simulink model "model_smpl"  (R2015a)
settings: Solver=ode45  StartTime=0.0  StopTime=Tfin  RelTol=1e-3
model workspace (MAT data in the model file):
  Sig = Simulink.Signal
  Sig.DataType = 'double'
  Sig.Dimensions = -1
  Sig.DimensionsMode = 'auto'
  Sig.Complexity = 'real'
  Sig.SampleTime = -1
  Sig.SamplingMode = 'auto'
  Sig.InitialValue = '[ ]'
values from neighbouring files (symbols this model uses):
  init_state = [ p_ini ]'    [main_parts.m]
  init_state_dot = [ 0 0 0 0 ]'    [main_parts.m]
undefined symbols (not defined in the file or in its folder): K, param, x, x_dot, x_r, y, y_dot, y_r
settings Model: Creator=jesus  LastModifiedBy=jesus

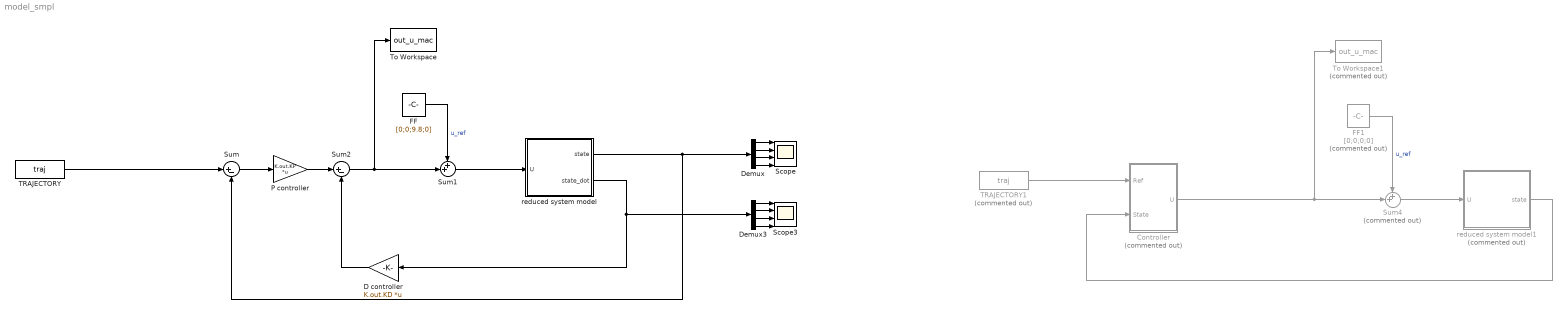
== system model_smpl ==
  Controller : Subsystem  Commented=on
  D controller : Gain  Gain=K.out.KD  Multiplication=Matrix(K*u)
  Demux : Demux
  Demux3 : Demux
  FF : Constant  Value=[0;0;9.8;0]
  FF1 : Constant  Commented=on  Value=[0;0;0;0]
  P controller : Gain  Gain=K.out.KP  Multiplication=Matrix(K*u)
  Scope : Scope  NumInputPorts=4
      settings: YMin=-5~-5~-5~-5  YMax=5~5~5~5
  Scope3 : Scope  NumInputPorts=4
      settings: YMin=-5~-5~-5~-5  YMax=5~5~5~5  SaveName=ScopeData3
  Sum : Sum  Inputs=|+-
  Sum1 : Sum  Inputs=++|
  Sum2 : Sum  Inputs=|+-
  Sum4 : Sum  Commented=on  Inputs=++|
  TRAJECTORY : FromWorkspace  VariableName=traj  SampleTime=param.hs  Interpolate=off  OutputAfterFinalValue=Setting to zero
  TRAJECTORY1 : FromWorkspace  Commented=on  VariableName=traj  SampleTime=param.hs  Interpolate=off  OutputAfterFinalValue=Setting to zero
  To Workspace : ToWorkspace  VariableName=out_u_mac  SaveFormat=Structure With Time  SampleTime=-1
  To Workspace1 : ToWorkspace  Commented=on  VariableName=out_u_mac  SaveFormat=Structure With Time  SampleTime=-1
  reduced system model : Subsystem
  reduced system model1 : Subsystem  Commented=on
  wires:
  Demux/1 -> Scope/1
  Demux/2 -> Scope/2
  Demux/3 -> Scope/3
  Demux/4 -> Scope/4
  Sum1/1 -> reduced system model/1(U)
  reduced system model/1(state) -> Sum/2, Demux/1
  FF/1 -> Sum1/1  "u_ref"
  Sum2/1 -> To Workspace/1, Sum1/2
  D controller/1 -> Sum2/2
  P controller/1 -> Sum2/1
  Sum/1 -> P controller/1
  TRAJECTORY/1 -> Sum/1
  Demux3/1 -> Scope3/1
  Demux3/2 -> Scope3/2
  Demux3/3 -> Scope3/3
  Demux3/4 -> Scope3/4
  reduced system model/2(state_dot) -> D controller/1, Demux3/1
  Sum4/1 -> reduced system model1/1(U)
  FF1/1 -> Sum4/1  "u_ref"
  TRAJECTORY1/1 -> Controller/1(Ref)
  reduced system model1/1(state) -> Controller/2(State)
  Controller/1(U) -> To Workspace1/1, Sum4/2

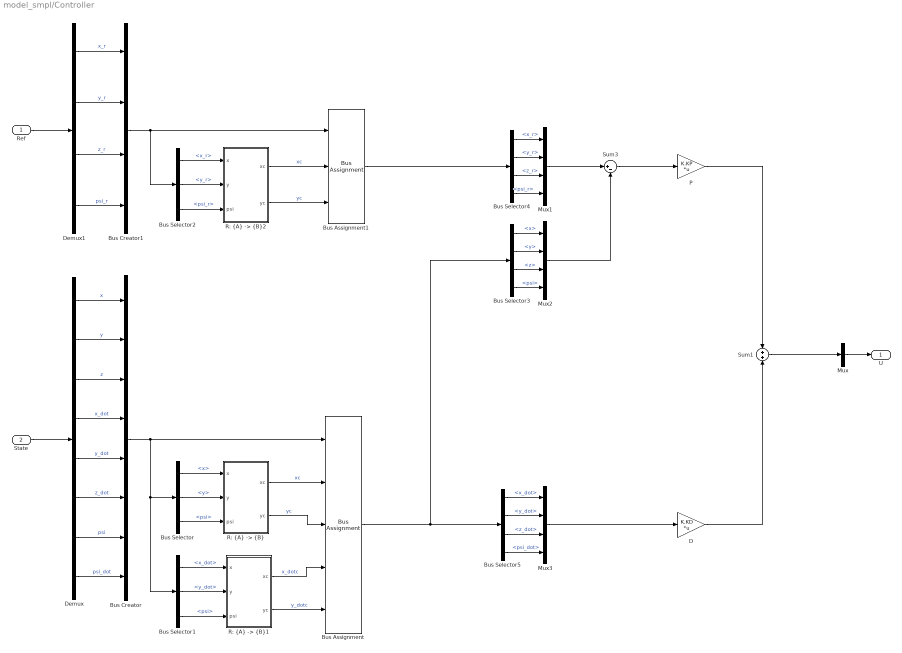
== system model_smpl/Controller ==
  Ref : Inport
  State : Inport  Port=2
  Bus Assignment : BusAssignment  AssignedSignals=x,y,x_dot,y_dot
  Bus Assignment1 : BusAssignment  AssignedSignals=x_r,y_r
  Bus Creator : BusCreator  Inputs=8
  Bus Creator1 : BusCreator
  Bus Selector : BusSelector  OutputSignals=x,y,psi
  Bus Selector1 : BusSelector  OutputSignals=x_dot,y_dot,psi
  Bus Selector2 : BusSelector  OutputSignals=x_r,y_r,psi_r
  Bus Selector3 : BusSelector  OutputSignals=x,y,z,psi
  Bus Selector4 : BusSelector  OutputSignals=x_r,y_r,z_r,psi_r
  Bus Selector5 : BusSelector  OutputSignals=x_dot,y_dot,z_dot,psi_dot
  D : Gain  Gain=K.KD  Multiplication=Matrix(K*u)
  Demux : Demux  Outputs=8
  Demux1 : Demux
  Mux : Mux  Inputs=1
  Mux1 : Mux
  Mux2 : Mux
  Mux3 : Mux
  P : Gain  Gain=K.KP  Multiplication=Matrix(K*u)
  "R: {A} -> {B}" : MATLAB Function  TreatAsAtomicUnit=on
  "R: {A} -> {B}1" : MATLAB Function  TreatAsAtomicUnit=on
  "R: {A} -> {B}2" : MATLAB Function  TreatAsAtomicUnit=on
  Sum1 : Sum  Inputs=+|+
  Sum3 : Sum  Inputs=|+-
  U : Outport
  wires:
  Demux/1 -> Bus Creator/1  "x"
  Demux/2 -> Bus Creator/2  "y"
  Demux/3 -> Bus Creator/3  "z"
  Demux/4 -> Bus Creator/4  "x_dot"
  Demux/5 -> Bus Creator/5  "y_dot"
  Demux/6 -> Bus Creator/6  "z_dot"
  Demux/7 -> Bus Creator/7  "psi"
  Bus Selector/1 -> "R: {A} -> {B}"/1(x)  "<x>"
  Bus Selector/2 -> "R: {A} -> {B}"/2(y)  "<y>"
  Bus Selector/3 -> "R: {A} -> {B}"/3(psi)  "<psi>"
  "R: {A} -> {B}"/1(xc) -> Bus Assignment/2  "xc"
  "R: {A} -> {B}"/2(yc) -> Bus Assignment/3  "yc"
  Bus Creator/1 -> Bus Assignment/1, Bus Selector/1, Bus Selector1/1
  Bus Selector1/1 -> "R: {A} -> {B}1"/1(x)  "<x_dot>"
  Bus Selector1/2 -> "R: {A} -> {B}1"/2(y)  "<y_dot>"
  Bus Selector1/3 -> "R: {A} -> {B}1"/3(psi)  "<psi>"
  "R: {A} -> {B}1"/1(xc) -> Bus Assignment/4  "x_dotc"
  "R: {A} -> {B}1"/2(yc) -> Bus Assignment/5  "y_dotc"
  Demux/8 -> Bus Creator/8  "psi_dot"
  Ref/1 -> Demux1/1
  State/1 -> Demux/1
  Demux1/4 -> Bus Creator1/4  "psi_r"
  Demux1/1 -> Bus Creator1/1  "x_r"
  Demux1/2 -> Bus Creator1/2  "y_r"
  Demux1/3 -> Bus Creator1/3  "z_r"
  Bus Selector2/1 -> "R: {A} -> {B}2"/1(x)  "<x_r>"
  Bus Selector2/2 -> "R: {A} -> {B}2"/2(y)  "<y_r>"
  Bus Selector2/3 -> "R: {A} -> {B}2"/3(psi)  "<psi_r>"
  "R: {A} -> {B}2"/1(xc) -> Bus Assignment1/2  "xc"
  "R: {A} -> {B}2"/2(yc) -> Bus Assignment1/3  "yc"
  Bus Creator1/1 -> Bus Selector2/1, Bus Assignment1/1
  Bus Assignment1/1 -> Bus Selector4/1
  Bus Assignment/1 -> Bus Selector5/1, Bus Selector3/1
  Bus Selector3/2 -> Mux2/2  "<y>"
  Bus Selector3/1 -> Mux2/1  "<x>"
  Bus Selector4/3 -> Mux1/3  "<z_r>"
  Bus Selector4/2 -> Mux1/2  "<y_r>"
  Bus Selector4/1 -> Mux1/1  "<x_r>"
  Mux2/1 -> Sum3/2
  Mux1/1 -> Sum3/1
  Sum3/1 -> P/1
  Bus Selector4/4 -> Mux1/4  "<psi_r>"
  Bus Selector3/4 -> Mux2/4  "<psi>"
  Bus Selector3/3 -> Mux2/3  "<z>"
  Bus Selector5/4 -> Mux3/4  "<psi_dot>"
  Bus Selector5/3 -> Mux3/3  "<z_dot>"
  Bus Selector5/2 -> Mux3/2  "<y_dot>"
  Bus Selector5/1 -> Mux3/1  "<x_dot>"
  Mux3/1 -> D/1
  Mux/1 -> U/1
  D/1 -> Sum1/2
  P/1 -> Sum1/1
  Sum1/1 -> Mux/1

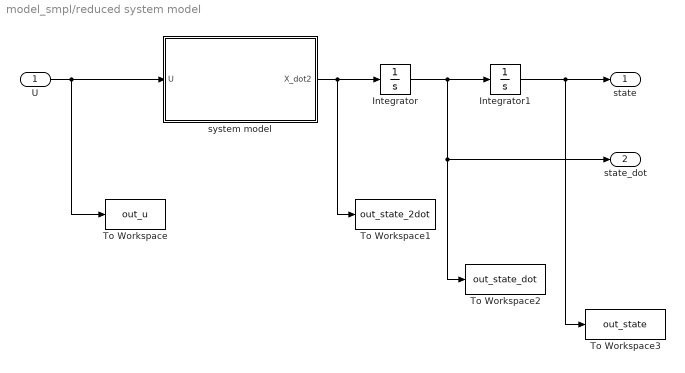
== system model_smpl/reduced system model ==
  U : Inport
  Integrator : Integrator  InitialCondition=init_state_dot
  Integrator1 : Integrator  InitialCondition=init_state
  To Workspace : ToWorkspace  VariableName=out_u  SaveFormat=Structure With Time  SampleTime=-1
  To Workspace1 : ToWorkspace  VariableName=out_state_2dot  SaveFormat=Structure With Time  SampleTime=-1
  To Workspace2 : ToWorkspace  VariableName=out_state_dot  SaveFormat=Structure With Time  SampleTime=-1
  To Workspace3 : ToWorkspace  VariableName=out_state  SaveFormat=Structure With Time  SampleTime=-1
  system model : MATLAB Function  TreatAsAtomicUnit=on
  state : Outport
  state_dot : Outport  Port=2
  wires:
  U/1 -> To Workspace/1, system model/1(U)
  Integrator/1 -> state_dot/1, To Workspace2/1, Integrator1/1
  system model/1(X_dot2) -> To Workspace1/1, Integrator/1
  Integrator1/1 -> To Workspace3/1, state/1

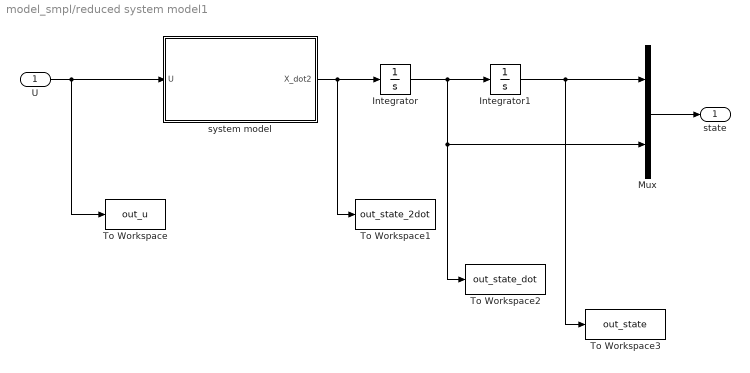
== system model_smpl/reduced system model1 ==
  U : Inport
  Integrator : Integrator  InitialCondition=init_state_dot
  Integrator1 : Integrator  InitialCondition=init_state
  Mux : Mux  Inputs=2
  To Workspace : ToWorkspace  VariableName=out_u  SaveFormat=Structure With Time  SampleTime=-1
  To Workspace1 : ToWorkspace  VariableName=out_state_2dot  SaveFormat=Structure With Time  SampleTime=-1
  To Workspace2 : ToWorkspace  VariableName=out_state_dot  SaveFormat=Structure With Time  SampleTime=-1
  To Workspace3 : ToWorkspace  VariableName=out_state  SaveFormat=Structure With Time  SampleTime=-1
  system model : MATLAB Function  TreatAsAtomicUnit=on
  state : Outport
  wires:
  U/1 -> To Workspace/1, system model/1(U)
  Integrator/1 -> Mux/2, To Workspace2/1, Integrator1/1
  system model/1(X_dot2) -> To Workspace1/1, Integrator/1
  Integrator1/1 -> Mux/1, To Workspace3/1
  Mux/1 -> state/1

== matlab function model_smpl/reduced system model1/system model ==
  data: U input; X_dot2 output
function X_dot2 = system(U)
% Simplified model of quadcopter
    % Inputs: F, Tpsi
    %   ·F: vector of forces in base{A}. projection of Thrust {B} in each
    %     direction of {A}
    %       units: [N]
    %   ·Tpsi: Torque applied around Euler's angle PSI
    %       units: [Nm]   
    %
    % Outputs: X_dot2: second derivative of the state
    %       units: ['state'/t^2]
    %
    % State: [x, y, z, psi]
    %       units: ['state']

% parameters
     m = 0.429;    g = 9.80665;   Iz = 0.00480374;

% MODEL
%   X_dot2 = (Mass, Inertia)*(F, Tpsi) + gravity
%   
A = diag([1/m 1/m 1/m 1/Iz]);

X_dot2 = A*U + [0; 0; 0; 0];

== matlab function model_smpl/reduced system model/system model ==
  data: U input; X_dot2 output
function X_dot2 = syst(U)
% Simplified model of quadcopter
    % Inputs: F, Tpsi
    %   ·F: vector of forces in base{A}. projection of Thrust {B} in each
    %     direction of {A}
    %       units: [N]
    %   ·Tpsi: Torque applied around Euler's angle PSI
    %       units: [Nm]   
    %
    % Outputs: X_dot2: second derivative of the state
    %       units: ['state'/t^2]
    %
    % State: [x, y, z, psi]
    %       units: ['state']

% parameters
     m = 0.429;    g = 9.80665;   Iz = 0.00480374;

% MODEL
%   X_dot2 = (1/Mass, 1/Inertia)*(F, Tpsi) + gravity
%   
A = diag([1/m 1/m 1/m 1/Iz]);

X_dot2 = A*U + [0; 0; -9.8; 0];

== matlab function model_smpl/Controller/R: {A} -> {B}2 ==
  data: x input; y input; psi input; xc output; yc output
function [xc, yc] = fcn(x, y, psi)
%#codegen
% Change in cordenates from fixed frame {A} to body frame {B} of position
%  state coordenates
% · apply rotation matrix over phi (vertical) to [x] and [y]
% · the references are given in fix frame {A}, input [u] is computed in
%   body frame {B}

R = [ cos(psi) sin(psi)
     -sin(psi) cos(psi)];
a = R * [x, y]';
xc = a(1);
yc = a(2);

== matlab function model_smpl/Controller/R: {A} -> {B} ==
  data: x input; y input; psi input; xc output; yc output
function [xc, yc] = fcn(x, y, psi)
%#codegen
% Change in cordenates from fixed frame {A} to body frame {B} of position
%  state coordenates
% · apply rotation matrix over phi (vertical) to [x] and [y]
% · the references are given in fix frame {A}, input [u] is computed in
%   body frame {B}

R = [ cos(psi) sin(psi)
     -sin(psi) cos(psi)];
a = R * [x, y]';
xc = a(1);
yc = a(2);

== matlab function model_smpl/Controller/R: {A} -> {B}1 ==
  data: x input; y input; psi input; xc output; yc output
function [xc, yc] = fcn(x, y, psi)
%#codegen
% Change in cordenates from fixed frame {A} to body frame {B} of position
%  state coordenates
% · apply rotation matrix over phi (vertical) to [x] and [y]
% · the references are given in fix frame {A}, input [u] is computed in
%   body frame {B}

R = [ cos(psi) sin(psi)
     -sin(psi) cos(psi)];
a = R * [x; y];
xc = a(1); 
yc = a(2);
